simulink subsystem "Motor_sub"  (R2023b)
settings: Solver=VariableStepAuto  StartTime=0.0  StopTime=10.0  RelTol=1e-3
libraries: arduinolib x6, simulink x2
settings Model: Creator=alumnos  LastModifiedBy=Usuario_UMA

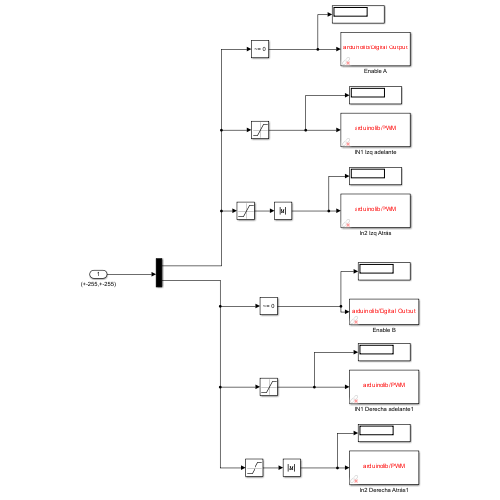
[thumbnail: Simulink's stored preview of the top-level diagram]
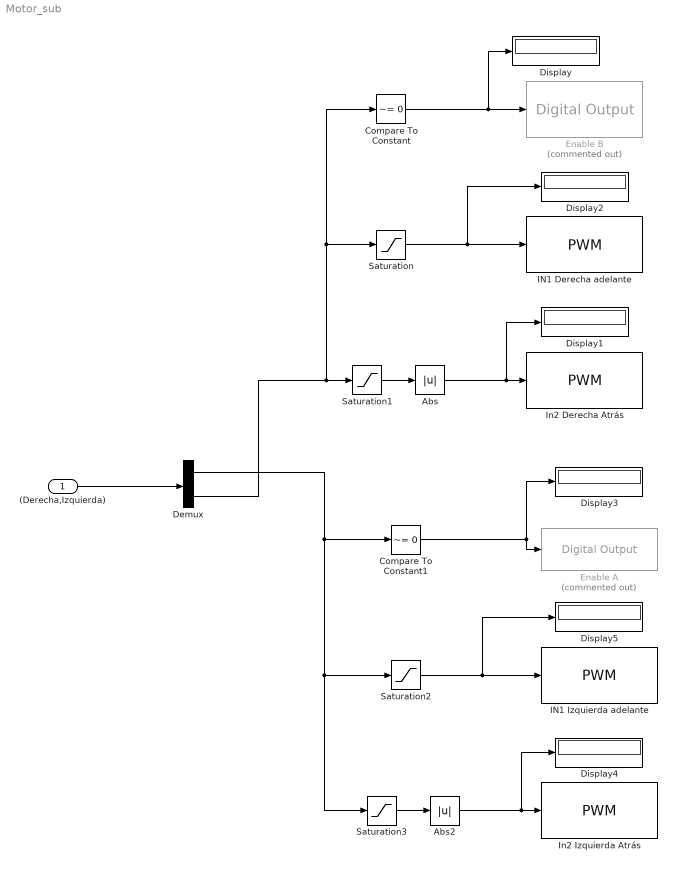
== system Motor_sub ==
  (Derecha,Izquierda) : Inport
  Abs : Abs  SaturateOnIntegerOverflow=off
  Abs2 : Abs  SaturateOnIntegerOverflow=off
  Compare To Constant : simulink/Logic and Bit Operations/Compare To Constant  relop=~=  const=0  OutDataTypeStr=boolean
  Compare To Constant1 : simulink/Logic and Bit Operations/Compare To Constant  relop=~=  const=0  OutDataTypeStr=boolean
  Demux : Demux  Outputs=2
  Display{,1..5} (6 alike) : Display
  Enable A : arduinolib/Digital Output  Commented=on  pinNumber=8  Direction=output  blockPlatform=arduino
  Enable B : arduinolib/Digital Output  Commented=on  pinNumber=9  Direction=output  blockPlatform=arduino
  IN1 Derecha adelante : arduinolib/PWM  pinNumber=11  frequencyType=Default  desiredFrequency=490.2  achievableFrequency=490.2
  IN1 Izquierda adelante : arduinolib/PWM  pinNumber=9  frequencyType=Default  desiredFrequency=490.2  achievableFrequency=490.2
  In2 Derecha Atrás : arduinolib/PWM  pinNumber=12  frequencyType=Default  desiredFrequency=490.2  achievableFrequency=490.2
  In2 Izquierda Atrás : arduinolib/PWM  pinNumber=10  frequencyType=Default  desiredFrequency=490.2  achievableFrequency=490.2
  Saturation : Saturate  UpperLimit=255  LowerLimit=0
  Saturation1 : Saturate  UpperLimit=0  LowerLimit=-255
  Saturation2 : Saturate  UpperLimit=255  LowerLimit=0
  Saturation3 : Saturate  UpperLimit=0  LowerLimit=-255
  wires:
  (Derecha,Izquierda)/1 -> Demux/1
  Saturation3/1 -> Abs2/1
  Abs2/1 -> Display4/1, In2 Izquierda Atrás/1
  Compare To Constant1/1 -> Display3/1, Enable A/1
  Compare To Constant/1 -> Display/1, Enable B/1
  Saturation1/1 -> Abs/1
  Abs/1 -> Display1/1, In2 Derecha Atrás/1
  Demux/2 -> Saturation/1, Compare To Constant/1, Saturation1/1
  Saturation2/1 -> Display5/1, IN1 Izquierda adelante/1
  Saturation/1 -> Display2/1, IN1 Derecha adelante/1
  Demux/1 -> Compare To Constant1/1, Saturation2/1, Saturation3/1
